simulink model "joystick"  (R2021b)
settings: Solver=FixedStepAuto  StartTime=0.0  StopTime=inf  FixedStep=0.1  RelTol=1e-3
InitFcn:
  | %for the case the code is run from the simulink folder
  |  %for the case run from the git root
  | addpath(genpath(pwd))
  | %for the case run simulink
  | folder=cd;
  | folder=fullfile(folder, '..');
  | addpath(genpath(folder)) %for the case run from the git root
  | %initialize the model
  | init
settings Model: Creator=ErikWilhelm  LastModifiedBy=ErikWilhelm

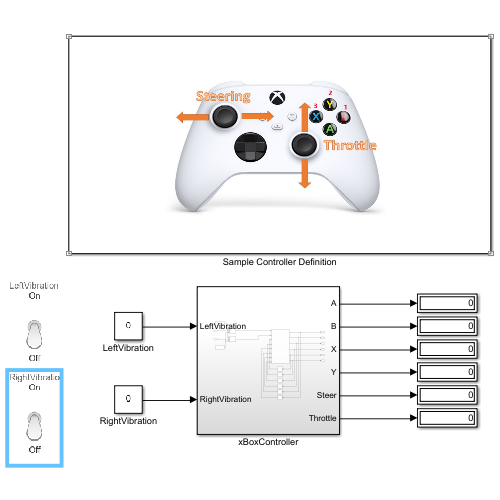
[thumbnail: Simulink's stored preview of the top-level diagram]
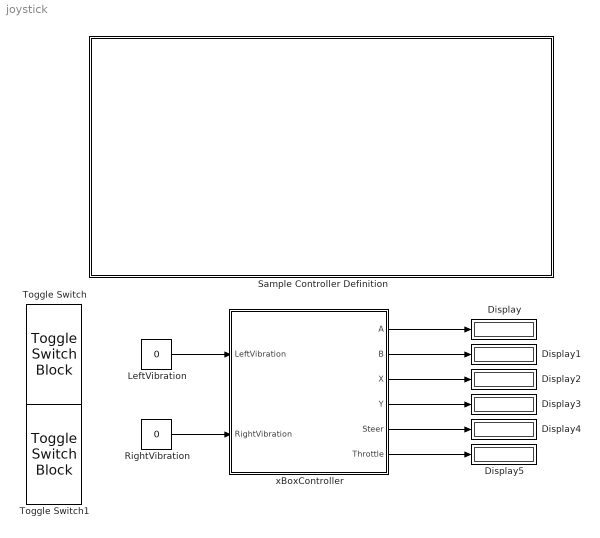
== system joystick ==
  Display{,1..5} (6 alike) : Display
  LeftVibration : Constant  Value=0  OutDataTypeStr=boolean
  RightVibration : Constant  Value=0  OutDataTypeStr=boolean
  Sample Controller Definition : Subsystem  RequirementInfo={} %GIDa_6afd2599_d1a7_4adc_9889_53d3a46ba436
      mask Display: image('C:\Users\ErikWilhelm\Documents\GitHub\Simulink_Xbox_Joystick\Resources\Controller_defn.jpg'); % Use "Edit Image" on toolstrip to change.
  Toggle Switch : ToggleSwitchBlock
      settings: Values={{'Off', 'On'}, [0 1]}
  Toggle Switch1 : ToggleSwitchBlock
      settings: Values={{'Off', 'On'}, [0 1]}
  xBoxController : Subsystem
  wires:
  xBoxController/1(A) -> Display/1
  xBoxController/2(B) -> Display1/1
  xBoxController/3(X) -> Display2/1
  xBoxController/4(Y) -> Display3/1
  xBoxController/5(Steer) -> Display4/1
  RightVibration/1 -> xBoxController/2(RightVibration)
  LeftVibration/1 -> xBoxController/1(LeftVibration)
  xBoxController/6(Throttle) -> Display5/1

== system joystick/Sample Controller Definition ==

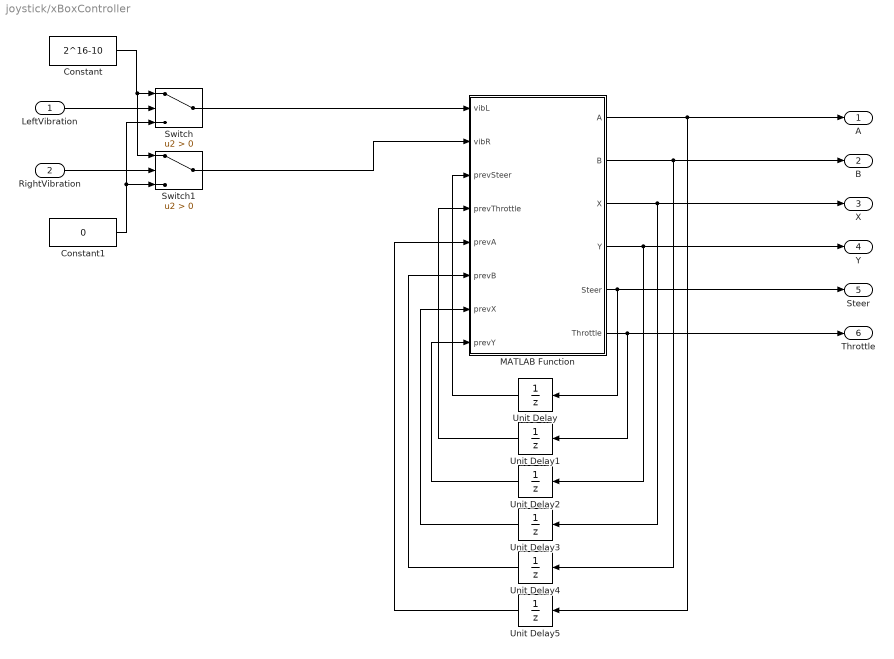
== system joystick/xBoxController ==
  LeftVibration : Inport
  RightVibration : Inport  Port=2
  Constant : Constant  Value=2^16-10
  Constant1 : Constant  Value=0
  MATLAB Function : MATLAB Function  TreatAsAtomicUnit=on
  Switch : Switch  Criteria=u2 > Threshold
  Switch1 : Switch  Criteria=u2 > Threshold
  Unit Delay{,1..5} (6 alike) : UnitDelay  SampleTime=-1  HasFrameUpgradeWarning=on
  A : Outport
  B : Outport  Port=2
  X : Outport  Port=3
  Y : Outport  Port=4
  Steer : Outport  Port=5
  Throttle : Outport  Port=6
  wires:
  Unit Delay5/1 -> MATLAB Function/5(prevA)
  Unit Delay4/1 -> MATLAB Function/6(prevB)
  Unit Delay3/1 -> MATLAB Function/7(prevX)
  Unit Delay2/1 -> MATLAB Function/8(prevY)
  Switch1/1 -> MATLAB Function/2(vibR)
  Constant1/1 -> Switch1/3, Switch/3
  Constant/1 -> Switch/1, Switch1/1
  Switch/1 -> MATLAB Function/1(vibL)
  RightVibration/1 -> Switch1/2
  LeftVibration/1 -> Switch/2
  Unit Delay1/1 -> MATLAB Function/4(prevThrottle)
  Unit Delay/1 -> MATLAB Function/3(prevSteer)
  MATLAB Function/6(Throttle) -> Unit Delay1/1, Throttle/1
  MATLAB Function/5(Steer) -> Unit Delay/1, Steer/1
  MATLAB Function/4(Y) -> Y/1, Unit Delay2/1
  MATLAB Function/3(X) -> X/1, Unit Delay3/1
  MATLAB Function/2(B) -> B/1, Unit Delay4/1
  MATLAB Function/1(A) -> A/1, Unit Delay5/1

== matlab function joystick/xBoxController/MATLAB Function ==
  data: vibL input; A output; vibR input; prevSteer input; prevThrottle input; B output; X output; Y output; Steer output; Throttle output; prevA input; prevB input; prevX input; prevY input
function [A,B,X,Y,Steer,Throttle] = PythonJoystickWrapper(vibL,vibR,prevSteer,prevThrottle,prevA,prevB,prevX,prevY)
    A=prevA;
    B=prevB;
    X=prevX;
    Y=prevY;
    Steer=prevSteer;
    Throttle=prevThrottle;
    vars= {0,0,0,0,0,0};
    coder.extrinsic('py.SimJoystick.ev')
    output=py.SimJoystick.ev(vibL,vibR,prevSteer,prevThrottle,prevA,prevB,prevX,prevY);
    vars=cell(output);
    A=vars{1};
    B=vars{2};
    X=vars{3};
    Y=vars{4};
    Steer=vars{5};
    Throttle=vars{6};
end
